simulink model "R0005E_Tanksim"  (R2020a)
settings: Solver=ode5  StartTime=0.0  StopTime=300  RelTol=1e-3  EnableMultiTasking=on
undefined symbols (not defined in the file): A1, a1, A2, a2
libraries: R0005E_lib x1
settings Model: Creator=wolfgang  LastModifiedBy=Wolfgang
settings Model: ModifiedHistory=|
  | Created an adjusted empty Simulink diagram for the lab assignments
  | in the course R0002E
settings DataIOCC: SaveFormat=Array  SignalLoggingSaveFormat=ModelDataLogs  SaveOutput=off  SignalLogging=off  DSMLogging=off  SaveTime=off  ReturnWorkspaceOutputs=off
settings OptimizationCC: ExpressionDepthLimit=2147483647  LifeSpan=inf
settings DebuggingCC: UnderspecifiedInitializationDetection=Classic  MergeDetectMultiDrivingBlocksExec=none  SolverPrmCheckMsg=warning  FcnCallInpInsideContextMsg=warning  StateNameClashWarn=warning  SFUnexpectedBacktrackingDiag=warning  SFNoUnconditionalDefaultTransitionDiag=warning  SFExecutionAtInitializationDiag=none  ArithmeticOperatorsInVariantConditions=warning
settings HardwareCC: ProdBitPerPointer=32  ProdBitPerSizeT=32  ProdBitPerPtrDiffT=32  ProdLargestAtomicFloat=None  ProdIntDivRoundTo=Undefined  ProdEndianess=Unspecified  ProdWordSize=32  ProdHWDeviceType=32-bit Generic
settings ModelReferenceCC: PropagateSignalLabelsOutOfModel=off
settings SFSimCC: SimUseLocalCustomCode=off  CustomCodeUndefinedFunction=UseInterfaceOnly
settings RTWCC: RTWUseLocalCustomCode=off
settings CodeAppCC: StateflowObjectComments=on
settings GRTTargetCC: TargetLangStandard=C89/C90 (ANSI)
settings ConfigComp: CovMetricSettings=dw  CovHtmlReporting=on  CovSaveCumulativeToWorkspaceVar=on  CovSaveSingleToWorkspaceVar=on  CovExternalEMLEnable=off

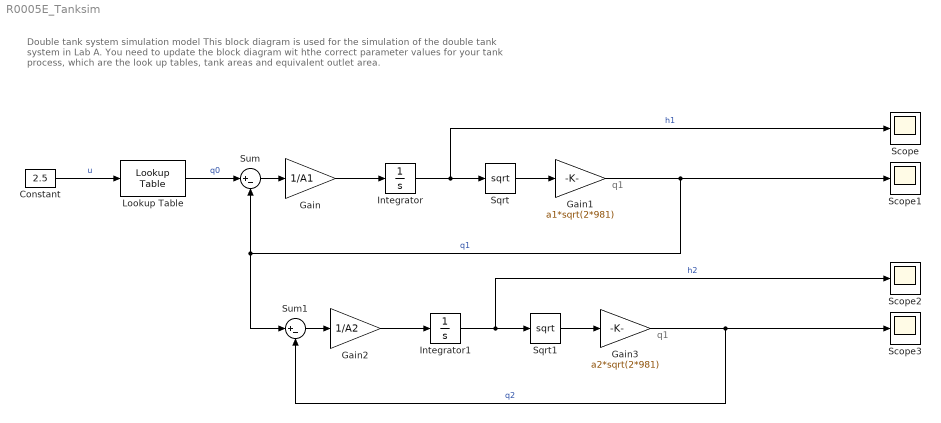
== system R0005E_Tanksim ==
  note: Double tank system simulation model
      |
      | This block diagram is used for the simulation of the double tank system in Lab A.
      | You need to update the block diagram wit hthe correct parameter
      | values for your tank process, which are the look up tables, tank areas and
      | equivalent outlet area.
  note: q1
  note: q1
  Constant : Constant  Value=2.5
  Gain : Gain  Gain=1/A1
  Gain1 : Gain  Gain=a1*sqrt(2*981)
  Gain2 : Gain  Gain=1/A2
  Gain3 : Gain  Gain=a2*sqrt(2*981)
  Integrator : Integrator
  Integrator1 : Integrator
  Lookup Table : R0005E_lib/Lookup Table  x=[0,1,2,3,4,5,6,7,8,9,10]  y=[0,3,4,5,7,8,9,11,12,15,16]
  Scope{,1..3} (4 alike) : Scope
  Sqrt : Sqrt  SaturateOnIntegerOverflow=on
  Sqrt1 : Sqrt  SaturateOnIntegerOverflow=on
  Sum : Sum  Inputs=|+-
  Sum1 : Sum  Inputs=|+-
  wires:
  Sum1/1 -> Gain2/1
  Gain2/1 -> Integrator1/1
  Sqrt1/1 -> Gain3/1
  Gain1/1 -> Sum1/1, Sum/2, Scope1/1  "q1"
  Gain3/1 -> Scope3/1, Sum1/2  "q2"
  Integrator/1 -> Sqrt/1, Scope/1  "h1"
  Integrator1/1 -> Scope2/1, Sqrt1/1  "h2"
  Lookup Table/1 -> Sum/1  "q0"
  Sum/1 -> Gain/1
  Constant/1 -> Lookup Table/1  "u"
  Gain/1 -> Integrator/1
  Sqrt/1 -> Gain1/1
